simulink model "qcm"  (R2017b)
settings: Solver=VariableStepAuto  StartTime=0.0  StopTime=5  RelTol=1e-3
values from neighbouring files (symbols this model uses):
  loc = 1    [init.m]
  qcm = struct(qcm)    [constants18.m]
  setV = 0    [init.m]
  your_dut = 18    [init.m]
  Zs0 = [0 0 0 0]    [constants18.m]
  Zu0 = [0 0 0 0]    [constants18.m]
undefined symbols (not defined in the file or in its folder): sigbuilder_block
libraries: simulink x1
settings Model: Creator=Aleksis  LastModifiedBy=rvorster
settings CodeAppCC: StateflowObjectComments=on

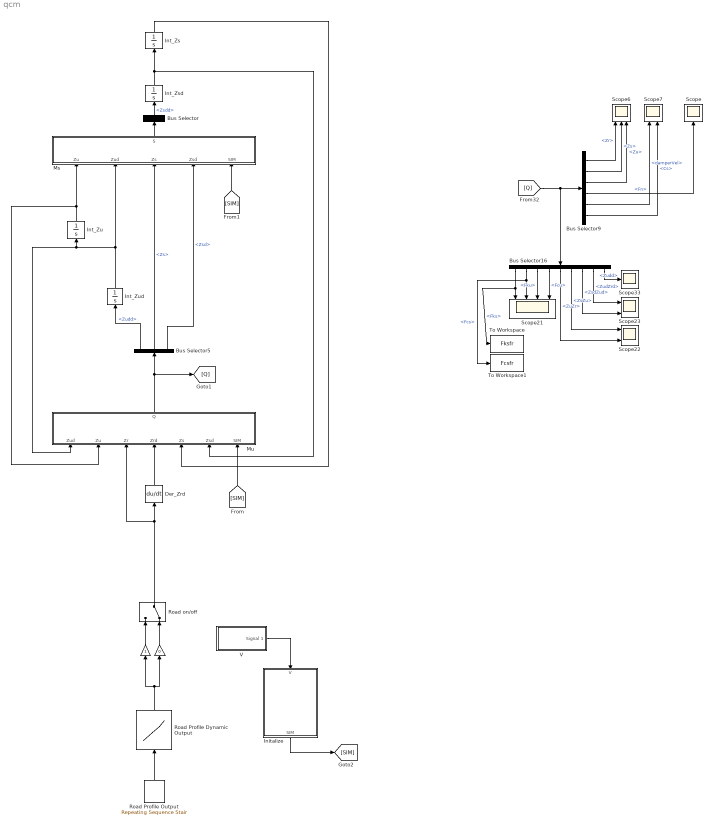
== system qcm ==
  " " : Gain
  " " : Gain  Gain=0
  Bus Selector : BusSelector  OutputSignals=Zsdd
  Bus Selector16 : BusSelector  OutputSignals=Fks,Fcs,Fku,Fcu,ZuZr,ZsZu,ZsdZud,ZudZrd,Zudd
  Bus Selector5 : BusSelector  OutputSignals=Zudd,Zs,Zsd
  Bus Selector9 : BusSelector  OutputSignals=Zr,Zs,Zu,Fn,damperVel,Cs
  Der_Zrd : Derivative
  Initalize : MATLAB Function  TreatAsAtomicUnit=on
  Int_Zs : Integrator  InitialCondition=-Zs0(1)
  Int_Zsd : Integrator
  Int_Zu : Integrator  InitialCondition=-Zu0(1)
  Int_Zud : Integrator
  Ms : MATLAB Function  TreatAsAtomicUnit=on
  Mu : MATLAB Function  TreatAsAtomicUnit=on
  Road Profile Dynamic Output : Lookup_n-D  NumberOfTableDimensions=1  BreakpointsForDimension1=[-5:5]  Table=tanh([-5:5])  InternalRulePriority=Speed  RndMeth=Simplest  InputSameDT=on
  Road Profile Output : simulink/Sources/Repeating Sequence Stair  OutValues=hx_left  tsamp=time_step  OutMin=[]  OutMax=[]  OutDataTypeStr=double  OutputDataTypeScalingMode=double  OutDataType=fixdt(0,8)  ConRadixGroup=Best Precision: Vector-wise  OutScaling=2^-12
  "Road on/off " : ManualSwitch  CurrentSetting=0
  Scope : Scope
  Scope21 : Scope  NumInputPorts=4
  Scope22 : Scope  NumInputPorts=2
  Scope23 : Scope  NumInputPorts=2
  Scope33 : Scope
  Scope6 : Scope  NumInputPorts=3
  Scope7 : Scope  NumInputPorts=2
  To Workspace : ToWorkspace  VariableName=Fksfr  SaveFormat=Timeseries  SampleTime=-1
  To Workspace1 : ToWorkspace  VariableName=Fcsfr  SaveFormat=Timeseries  SampleTime=-1
  V : Subsystem  Tag=STV Subsys  LoadFcn=sigbuilder_block('load');  StartFcn=sigbuilder_block('start');  StopFcn=sigbuilder_block('stop');  ClipboardFcn=sigbuilder_block('clipboard');  mask(Sigbuilder block){tuvar=[0:10]}
      mask help: Simulink:masks:SigbuilderBlock_MD
      mask init:
      | if ~strcmp(get_param(bdroot(gcbh),'SimulationStatus'),'stopped') tuvar = sigbuilder_block('maskInit'); end
      settings: CopyFcn=sigbuilder_block('copy');  DeleteFcn=sigbuilder_block('delete');  ModelCloseFcn=sigbuilder_block('modelClose');  PreSaveFcn=sigbuilder_block('preSave');  PauseFcn=sigbuilder_block('pause');  ContinueFcn=sigbuilder_block('continue');  NameChangeFcn=sigbuilder_block('namechange');  OpenFcn=sigbuilder_block('open',[433.5 195.75 558 401.25 ]);  CloseFcn=sigbuilder_block('close');
      mask Display: plot(0, 0, 100, 100,[2, 2, 32, 32, 2], [68, 8, 8, 68, 68],[32, 2], [38, 38], [32, 19, 2],[53, 60, 44], [32, 17, 17, 2],[16, 16, 31, 31]);txt = getActiveGroup(gcbh);text(2, 100, txt,'verticalAlignment', 'top');
  wires:
  "Road on/off "/1 -> Mu/3(Zr), Der_Zrd/1
  Der_Zrd/1 -> Mu/4(Zrd)
  Int_Zud/1 -> Mu/1(Zud), Int_Zu/1, Ms/2(Zud)
  Int_Zu/1 -> Mu/2(Zu), Ms/1(Zu)
  Int_Zsd/1 -> Mu/6(Zsd), Int_Zs/1
  Bus Selector5/2 -> Ms/3(Zs)  "<Zs>"
  Bus Selector5/3 -> Ms/4(Zsd)  "<Zsd>"
  Int_Zs/1 -> Mu/5(Zs)
  Road Profile Output/1 -> Road Profile Dynamic Output/1
  " "/1 -> "Road on/off "/2
  " "/1 -> "Road on/off "/1
  Road Profile Dynamic Output/1 -> " "/1, " "/1
  Mu/1(Q) -> [Q], Bus Selector5/1
  Bus Selector5/1 -> Int_Zud/1  "<Zudd>"
  V/1(Signal 1) -> Initalize/1(V)
  Initalize/1(SIM) -> [SIM]
  [SIM] -> Mu/7(SIM)
  [SIM] -> Ms/5(SIM)
  Bus Selector9/3 -> Scope6/3  "<Zu>"
  Bus Selector16/1 -> To Workspace/1, Scope21/1  "<Fks>"
  Bus Selector9/5 -> Scope7/1  "<damperVel>"
  Bus Selector16/8 -> Scope23/1  "<ZudZrd>"
  Bus Selector9/6 -> Scope7/2  "<Cs>"
  Bus Selector16/4 -> Scope21/4  "<Fcu>"
  Bus Selector16/7 -> Scope23/2  "<ZsdZud>"
  Bus Selector16/5 -> Scope22/2  "<ZuZr>"
  Bus Selector16/2 -> To Workspace1/1, Scope21/2  "<Fcs>"
  Bus Selector9/2 -> Scope6/2  "<Zs>"
  Bus Selector16/6 -> Scope22/1  "<ZsZu>"
  Bus Selector9/4 -> Scope/1  "<Fn>"
  Bus Selector16/3 -> Scope21/3  "<Fku>"
  Bus Selector16/9 -> Scope33/1  "<Zudd>"
  Bus Selector9/1 -> Scope6/1  "<Zr>"
  [Q] -> Bus Selector9/1, Bus Selector16/1
  Ms/1(S) -> Bus Selector/1
  Bus Selector/1 -> Int_Zsd/1  "<Zsdd>"

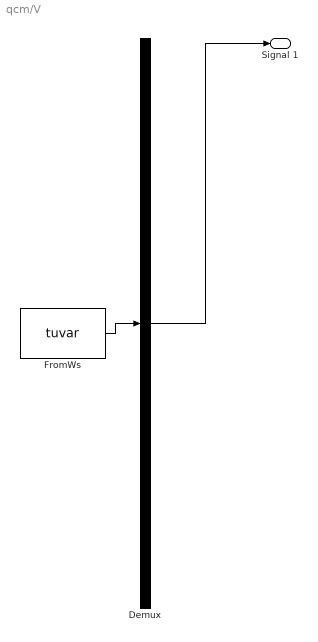
== system qcm/V ==
  Demux : Demux  Tag=STV Demux  Outputs=1
  FromWs : FromWorkspace  Tag=STV FromWs  VariableName=tuvar  SampleTime=0
      SigBuilderData=|
      | common.afterFinalStr = 'Extrapolate'
      | common.sampleTime = 0
      | dataSet.timeRange = [0 10]
      | dataSet.name = 'Group 1'
      | sbobj.Groups.Name = 'Group 1'
      | sbobj.Groups.Signals.Name = 'Signal 1'
      | sbobj.Groups.Signals.XData = [0 4 6 10]
      | sbobj.Groups.Signals.YData = [0 35 0 0]
  Signal 1 : Outport  Tag=STV Outport
  wires:
  Demux/1 -> Signal 1/1
  FromWs/1 -> Demux/1

== matlab function qcm/Ms ==
  data: Zu input; Zud input; Zs input; Zsd input; SIM input Bus: SIM; S output Bus: C; qcm parameter; loc parameter
function S = fcm(Zu, Zud, Zs, Zsd, SIM, qcm, loc)

    S = sprung_mass(Zu, Zud, Zs, Zsd, SIM, loc, qcm);
    
end

== matlab function qcm/Mu ==
  data: Zud input; Zu input; Zr input; Zrd input; Q output Bus: U; Zs input; Zsd input; qcm parameter; loc parameter; SIM input Bus: SIM; Zs0 parameter
function Q = fcn(Zud, Zu, Zr, Zrd, Zs, Zsd, qcm, loc, SIM, Zs0)

    Q = unsprung_mass(Zud, Zu, Zrd, Zr, Zsd, Zs, loc, SIM, Zs0, qcm);

end

== matlab function qcm/Initalize ==
  settings: updateMethod=DISCRETE
  data: V input; qcm parameter; SIM output Bus: SIM; setV parameter; loc parameter; your_dut parameter
function SIM = fcn(V, qcm, setV, loc, your_dut)

    if (setV == 0)
        SIM.V = qcm.V;
        SIM.L = 0.5*qcm.V^2*qcm.ClA*qcm.rho0;
        SIM.sim_time = 0;
        SIM.sim_step = 0;
        SIM.time_step = 0.01 / qcm.V;
        SIM.your_dut = your_dut;
        SIM.loc = loc;
    else
        SIM.V = V;
        SIM.L = 0.5*V^2*qcm.ClA*qcm.rho0;
        SIM.sim_time = 0;
        SIM.sim_step = 0;
        SIM.time_step = 0.01 / V;
        SIM.your_dut = your_dut;
        SIM.loc = loc;
    end

end
